simulink model "PSO_tunning_PID"  (R2019b)
settings: Solver=ode23s  StartTime=0.0  StopTime=10  RelTol=1000000
undefined symbols (not defined in the file or in its folder): xpid
libraries: simulink x3
settings Model: Creator=abdul  LastModifiedBy=ebunl
settings DataIOCC: SaveFormat=Array  ReturnWorkspaceOutputs=off
settings DebuggingCC: ArithmeticOperatorsInVariantConditions=warning
settings SFSimCC: SimUseLocalCustomCode=off  CustomCodeUndefinedFunction=UseInterfaceOnly
settings RTWCC: RTWUseLocalCustomCode=off
settings CodeAppCC: StateflowObjectComments=on

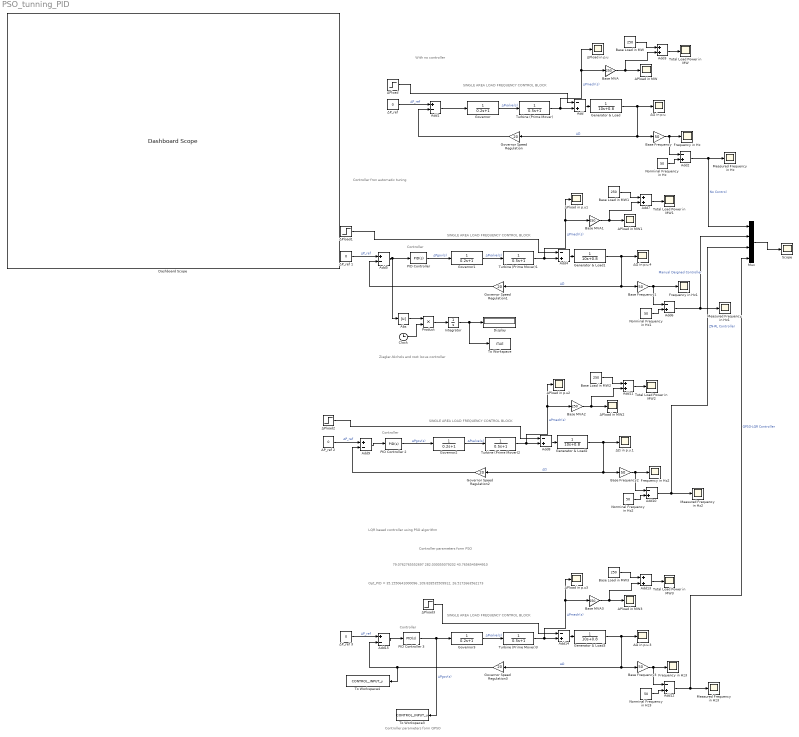
== system PSO_tunning_PID ==
  note: Opt_PID = 35.1550641000096 ,109.828535509912, 26.5172663562173
  note: Controller parameters form PSO
  note: 79.0762765552697 282.030055079202 43.7656545844910
  note: With no controller
  note: Controller
  note: SINGLE AREA LOAD FREQUENCY CONTROL BLOCK
  note: SINGLE AREA LOAD FREQUENCY CONTROL BLOCK
  note: SINGLE AREA LOAD FREQUENCY CONTROL BLOCK
  note: Controller
  note: Controller fron automatic tuning
  note: Ziegler-Nichols and root locus controller
  note: SINGLE AREA LOAD FREQUENCY CONTROL BLOCK
  note: Controller
  note: LQR based controller using PSO algorithm
  note: Controller parameters form QPSO
   Base Load in MW{,1..3} (4 alike) : Constant  Value=250
   Norminal Frequency in Hz{,1..3} (4 alike) : Constant  Value=50
  Abs : Abs
  Add{,2,4,6,8,10,12,14} (8 alike) : Sum  Inputs=-+
  Add{1,5,9,15} (4 alike) : Sum  Inputs=+-
  Add{3,7,11,13} (4 alike) : Sum
  Base Frequency{,1..3} (4 alike) : Gain  Gain=50
  Base MVA{,1..3} (4 alike) : Gain  Gain=250
  Clock : Clock
  Dashboard Scope : DashboardScope
  Display : Display
  Frequency in Hz{,1..3} (4 alike) : Scope
  Generator & Load{,1..3} (4 alike) : TransferFcn  Denominator=[10 0.8]
  Governor{,1..3} (4 alike) : TransferFcn  Denominator=[0.2 1]
  Governor Speed Regulation{,1..3} (4 alike) : Gain  Gain=20
  Integrator : Integrator
  Measured Frequency in Hz{,1..3} (4 alike) : Scope
  Mux : Mux
  "PID Controller " : simulink/Continuous/PID Controller  Controller=PID  Form=Parallel  TimeDomain=Continuous-time  SampleTime=-1  IntegratorMethod=Forward Euler  FilterMethod=Forward Euler  ControllerParametersSource=internal  P=2.0121  I=0.9989  D=1.0117  UseFilter=on  N=100  TunerSelectOption=Transfer Function Based (PID Tuner App)  InitialConditionSource=internal  InitialConditionForIntegrator=0  InitialConditionForFilter=0  DifferentiatorICPrevScaledInput=0  ExternalReset=none  TrackingMode=off  Kt=1  LimitOutput=off  UpperSaturationLimit=inf  LowerSaturationLimit=-inf  LinearizeAsGain=on  AntiWindupMode=none  Kb=1  POutMin=[]  POutMax=[]  IOutMin=[]  IOutMax=[]  DOutMin=[]  DOutMax=[]  NOutMin=[]  NOutMax=[]  SumOutMin=[]  SumOutMax=[]  SaturationOutMin=[]  SaturationOutMax=[]  PParamMin=[]  PParamMax=[]  IParamMin=[]  IParamMax=[]  DParamMin=[]  DParamMax=[]  NParamMin=[]  NParamMax=[]  KbParamMin=[]  KbParamMax=[]  KtParamMin=[]  KtParamMax=[]  KbOutMin=[]  KbOutMax=[]  KtOutMin=[]  KtOutMax=[]  IntegratorOutMin=[]  IntegratorOutMax=[]  FilterOutMin=[]  FilterOutMax=[]  SumI1OutMin=[]  SumI1OutMax=[]  SumI2OutMin=[]  SumI2OutMax=[]  SumI3OutMin=[]  SumI3OutMax=[]  SumI4OutMin=[]  SumI4OutMax=[]  SumDOutMin=[]  SumDOutMax=[]  DifferentiatorOutMin=[]  DifferentiatorOutMax=[]  FilterDiffOutCoefMin=[]  FilterDiffOutCoefMax=[]  ReciprocalOutMin=[]  ReciprocalOutMax=[]  SumDenOutMin=[]  SumDenOutMax=[]  SumNumOutMin=[]  SumNumOutMax=[]  DivideOutMin=[]  DivideOutMax=[]  IntegratorContinuousStateAttributes=''  IntegratorStateMustResolveToSignalObject=off  IntegratorRTWStateStorageClass=Auto  FilterContinuousStateAttributes=''  FilterStateMustResolveToSignalObject=off  FilterRTWStateStorageClass=Auto  ParallelPVariant=InternalParameters  IdealPVariant=Disabled  IVariant=InternalParameters  DVariant=InternalParameters  IntegratorVariant=Continuous  SatVariant=Disabled  AWVariant=Passthrough  PCopyVariant=Disabled  TRVariant=Disabled  FdbkBlocksVariant=Forward  IdealPFdbkVariant=Disabled  SatFdbkVariant=Disabled  DerivativeFilterVariant=ContFilter  NVariant=InternalParameters  NCopyVariant=Disabled  FilterICVariant=InternalICsFilter  IntegratorICVariant=InternalICs  ExternalResetVariant=Disabled  TRSumVariant=Passthrough  SumFdbkVariant=Disabled  SumVariant=Sum_PID
  PID Controller 2 : simulink/Continuous/PID Controller  Controller=PID  Form=Parallel  TimeDomain=Continuous-time  SampleTime=-1  IntegratorMethod=Forward Euler  FilterMethod=Forward Euler  ControllerParametersSource=internal  P=2.244  I=2.31937984  D=0.5427675  UseFilter=on  N=100  TunerSelectOption=Transfer Function Based (PID Tuner App)  InitialConditionSource=internal  InitialConditionForIntegrator=0  InitialConditionForFilter=0  DifferentiatorICPrevScaledInput=0  ExternalReset=none  TrackingMode=off  Kt=1  LimitOutput=off  UpperSaturationLimit=inf  LowerSaturationLimit=-inf  LinearizeAsGain=on  AntiWindupMode=none  Kb=1  POutMin=[]  POutMax=[]  IOutMin=[]  IOutMax=[]  DOutMin=[]  DOutMax=[]  NOutMin=[]  NOutMax=[]  SumOutMin=[]  SumOutMax=[]  SaturationOutMin=[]  SaturationOutMax=[]  PParamMin=[]  PParamMax=[]  IParamMin=[]  IParamMax=[]  DParamMin=[]  DParamMax=[]  NParamMin=[]  NParamMax=[]  KbParamMin=[]  KbParamMax=[]  KtParamMin=[]  KtParamMax=[]  KbOutMin=[]  KbOutMax=[]  KtOutMin=[]  KtOutMax=[]  IntegratorOutMin=[]  IntegratorOutMax=[]  FilterOutMin=[]  FilterOutMax=[]  SumI1OutMin=[]  SumI1OutMax=[]  SumI2OutMin=[]  SumI2OutMax=[]  SumI3OutMin=[]  SumI3OutMax=[]  SumI4OutMin=[]  SumI4OutMax=[]  SumDOutMin=[]  SumDOutMax=[]  DifferentiatorOutMin=[]  DifferentiatorOutMax=[]  FilterDiffOutCoefMin=[]  FilterDiffOutCoefMax=[]  ReciprocalOutMin=[]  ReciprocalOutMax=[]  SumDenOutMin=[]  SumDenOutMax=[]  SumNumOutMin=[]  SumNumOutMax=[]  DivideOutMin=[]  DivideOutMax=[]  IntegratorContinuousStateAttributes=''  IntegratorStateMustResolveToSignalObject=off  IntegratorRTWStateStorageClass=Auto  FilterContinuousStateAttributes=''  FilterStateMustResolveToSignalObject=off  FilterRTWStateStorageClass=Auto  ParallelPVariant=InternalParameters  IdealPVariant=Disabled  IVariant=InternalParameters  DVariant=InternalParameters  IntegratorVariant=Continuous  SatVariant=Disabled  AWVariant=Passthrough  PCopyVariant=Disabled  TRVariant=Disabled  FdbkBlocksVariant=Forward  IdealPFdbkVariant=Disabled  SatFdbkVariant=Disabled  DerivativeFilterVariant=ContFilter  NVariant=InternalParameters  NCopyVariant=Disabled  FilterICVariant=InternalICsFilter  IntegratorICVariant=InternalICs  ExternalResetVariant=Disabled  TRSumVariant=Passthrough  SumFdbkVariant=Disabled  SumVariant=Sum_PID
  PID Controller 3 : simulink/Continuous/PID Controller  Controller=PID  Form=Parallel  TimeDomain=Continuous-time  SampleTime=-1  IntegratorMethod=Forward Euler  FilterMethod=Forward Euler  ControllerParametersSource=internal  P=xpid(1)  I=xpid(2)  D=xpid(3)  UseFilter=on  N=100  TunerSelectOption=Transfer Function Based (PID Tuner App)  InitialConditionSource=internal  InitialConditionForIntegrator=0  InitialConditionForFilter=0  DifferentiatorICPrevScaledInput=0  ExternalReset=none  TrackingMode=off  Kt=1  LimitOutput=off  UpperSaturationLimit=inf  LowerSaturationLimit=-inf  LinearizeAsGain=on  AntiWindupMode=none  Kb=1  POutMin=[]  POutMax=[]  IOutMin=[]  IOutMax=[]  DOutMin=[]  DOutMax=[]  NOutMin=[]  NOutMax=[]  SumOutMin=[]  SumOutMax=[]  SaturationOutMin=[]  SaturationOutMax=[]  PParamMin=[]  PParamMax=[]  IParamMin=[]  IParamMax=[]  DParamMin=[]  DParamMax=[]  NParamMin=[]  NParamMax=[]  KbParamMin=[]  KbParamMax=[]  KtParamMin=[]  KtParamMax=[]  KbOutMin=[]  KbOutMax=[]  KtOutMin=[]  KtOutMax=[]  IntegratorOutMin=[]  IntegratorOutMax=[]  FilterOutMin=[]  FilterOutMax=[]  SumI1OutMin=[]  SumI1OutMax=[]  SumI2OutMin=[]  SumI2OutMax=[]  SumI3OutMin=[]  SumI3OutMax=[]  SumI4OutMin=[]  SumI4OutMax=[]  SumDOutMin=[]  SumDOutMax=[]  DifferentiatorOutMin=[]  DifferentiatorOutMax=[]  FilterDiffOutCoefMin=[]  FilterDiffOutCoefMax=[]  ReciprocalOutMin=[]  ReciprocalOutMax=[]  SumDenOutMin=[]  SumDenOutMax=[]  SumNumOutMin=[]  SumNumOutMax=[]  DivideOutMin=[]  DivideOutMax=[]  IntegratorContinuousStateAttributes=''  IntegratorStateMustResolveToSignalObject=off  IntegratorRTWStateStorageClass=Auto  FilterContinuousStateAttributes=''  FilterStateMustResolveToSignalObject=off  FilterRTWStateStorageClass=Auto  ParallelPVariant=InternalParameters  IdealPVariant=Disabled  IVariant=InternalParameters  DVariant=InternalParameters  IntegratorVariant=Continuous  SatVariant=Disabled  AWVariant=Passthrough  PCopyVariant=Disabled  TRVariant=Disabled  FdbkBlocksVariant=Forward  IdealPFdbkVariant=Disabled  SatFdbkVariant=Disabled  DerivativeFilterVariant=ContFilter  NVariant=InternalParameters  NCopyVariant=Disabled  FilterICVariant=InternalICsFilter  IntegratorICVariant=InternalICs  ExternalResetVariant=Disabled  TRSumVariant=Passthrough  SumFdbkVariant=Disabled  SumVariant=Sum_PID
  Product : Product
  Scope : Scope
  To Workspace : ToWorkspace  VariableName=ITAE  SampleTime=-1
  To Workspace3 : ToWorkspace  VariableName=CONTROL_INPUT_u  SampleTime=-1
  To Workspace4 : ToWorkspace  VariableName=CONTROL_INPUT_y  SampleTime=-1
  Total Load Power in MW{,1..3} (4 alike) : Scope
  Turbine (Prime Mover){,1..3} (4 alike) : TransferFcn  Denominator=[0.5 1]
  ∆P_ref {,1..3} (4 alike) : Constant  Value=0
  ∆Pload : Step  Time=100  Before=0.2  After=0.2  SampleTime=0
  ∆Pload in MW{,1..3} (4 alike) : Scope
  ∆Pload in p.u{,1..3} (4 alike) : Scope
  ∆Pload1 : Step  Time=100  Before=0.2  After=0.2  SampleTime=1
  ∆Pload2 : Step  Time=100  Before=0.2  After=0.2  SampleTime=0
  ∆Pload3 : Step  Time=100  Before=0.8  After=0.2  SampleTime=0
  ∆Ω in p.u.{,1,3..4} (4 alike) : Scope
  wires:
  Governor/1 -> Turbine (Prime Mover)/1  "∆Pvalve(s)"
  Add/1 -> Generator & Load/1
  Turbine (Prime Mover)/1 -> ∆Pload in p.u/1, Base MVA/1, Add/2  "∆Pmech(s)"
  Generator & Load/1 -> Base Frequency/1, Governor Speed Regulation/1, ∆Ω in p.u./1  "∆Ω"
  Governor Speed Regulation/1 -> Add1/2
  "∆P_ref "/1 -> Add1/1  "∆P_ref"
  ∆Pload/1 -> Add/1
  Base Frequency/1 -> Add2/1, Frequency in Hz/1
  " Norminal Frequency in Hz"/1 -> Add2/2
  Add2/1 -> Mux/1, Measured Frequency in Hz/1  "No Control"
  Base MVA/1 -> Add3/2, ∆Pload in MW/1
  " Base Load in MW"/1 -> Add3/1
  Add3/1 -> Total Load Power in MW/1
  Add7/1 -> Total Load Power in MW1/1
  " Base Load in MW1"/1 -> Add7/1
  Base MVA1/1 -> ∆Pload in MW1/1, Add7/2
  Add6/1 -> Mux/2, Measured Frequency in Hz1/1  "Manual Deigned Controller"
  " Norminal Frequency in Hz1"/1 -> Add6/2
  Base Frequency1/1 -> Frequency in Hz1/1, Add6/1
  ∆Pload1/1 -> Add4/1
  Generator & Load1/1 -> ∆Ω in p.u.4/1, Governor Speed Regulation1/1, Base Frequency1/1  "∆Ω"
  Add5/1 -> "PID Controller "/1, Abs/1
  Turbine (Prime Mover)1/1 -> Add4/2, Base MVA1/1, ∆Pload in p.u1/1  "∆Pmech(s)"
  Add4/1 -> Generator & Load1/1
  Governor1/1 -> Turbine (Prime Mover)1/1  "∆Pvalve(s)"
  Abs/1 -> Product/1
  Clock/1 -> Product/2
  Product/1 -> Integrator/1
  Integrator/1 -> To Workspace/1, Display/1
  Governor Speed Regulation1/1 -> Add5/2
  ∆P_ref 1/1 -> Add5/1  "∆P_ref"
  Mux/1 -> Scope/1
  Turbine (Prime Mover)2/1 -> Add8/2, Base MVA2/1, ∆Pload in p.u2/1  "∆Pmech(s)"
  Governor Speed Regulation2/1 -> Add9/2
  Base MVA2/1 -> ∆Pload in MW2/1, Add11/2
  ∆P_ref 2/1 -> Add9/1  "∆P_ref"
  " Norminal Frequency in Hz2"/1 -> Add10/2
  PID Controller 2/1 -> Governor2/1  "∆Pgov(s)"
  Generator & Load2/1 -> ∆Ω in p.u.1/1, Governor Speed Regulation2/1, Base Frequency2/1  "∆Ω"
  Governor2/1 -> Turbine (Prime Mover)2/1  "∆Pvalve(s)"
  ∆Pload2/1 -> Add8/1
  Add10/1 -> Mux/3, Measured Frequency in Hz2/1  "ZN-RL Controller"
  Base Frequency2/1 -> Frequency in Hz2/1, Add10/1
  Add8/1 -> Generator & Load2/1
  Add9/1 -> PID Controller 2/1
  Add11/1 -> Total Load Power in MW2/1
  " Base Load in MW2"/1 -> Add11/1
  " Base Load in MW3"/1 -> Add13/1
  Add13/1 -> Total Load Power in MW3/1
  Add15/1 -> PID Controller 3/1
  Add14/1 -> Generator & Load3/1
  Base Frequency3/1 -> Frequency in Hz3/1, Add12/1
  Add12/1 -> Mux/4, Measured Frequency in Hz3/1  "QPSO-LQR Controller"
  ∆Pload3/1 -> Add14/1
  Governor3/1 -> Turbine (Prime Mover)3/1  "∆Pvalve(s)"
  Generator & Load3/1 -> Base Frequency3/1, Governor Speed Regulation3/1, ∆Ω in p.u.3/1  "∆Ω"
  PID Controller 3/1 -> Governor3/1, To Workspace3/1  "∆Pgov(s)"
  " Norminal Frequency in Hz3"/1 -> Add12/2
  ∆P_ref 3/1 -> Add15/1  "∆P_ref"
  Base MVA3/1 -> Add13/2, ∆Pload in MW3/1
  Governor Speed Regulation3/1 -> Add15/2, To Workspace4/1
  Turbine (Prime Mover)3/1 -> ∆Pload in p.u3/1, Base MVA3/1, Add14/2  "∆Pmech(s)"
  "PID Controller "/1 -> Governor1/1  "∆Pgov(s)"
  Add1/1 -> Governor/1
